simulink model "hw7_system"  (R2015a)
settings: Solver=ode3  StartTime=0.0  StopTime=20  FixedStep=.01  MaxStep=.01  MinStep=.01  RelTol=1e-3
settings Model: Creator=lbremer  LastModifiedBy=lbremer

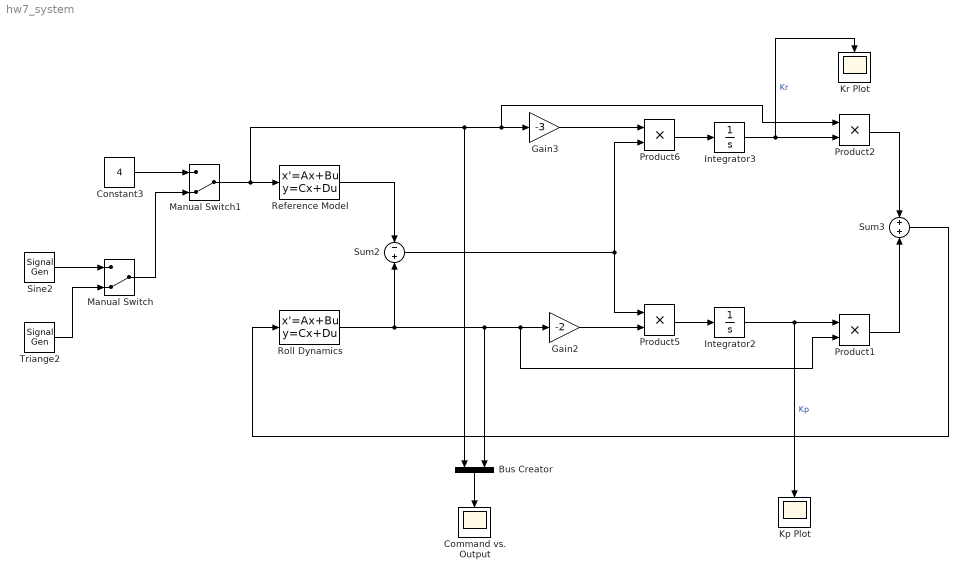
== system hw7_system ==
  Bus Creator : BusCreator  Inputs=2
  Command vs. Output : Scope
      settings: YMin=-1  YMax=1  SaveName=ScopeData4
  Constant3 : Constant  Value=4
  Gain2 : Gain  Gain=-2
  Gain3 : Gain  Gain=-3
  Integrator2 : Integrator
  Integrator3 : Integrator
  Kp Plot : Scope
      settings: YMin=-1  YMax=1
  "Kr Plot " : Scope
      settings: YMin=-1  YMax=1
  Manual Switch : ManualSwitch  CurrentSetting=0
  Manual Switch1 : ManualSwitch  CurrentSetting=0
  Product{1..2,5..6} (4 alike) : Product
  "Reference Model " : StateSpace  A=-6  B=6  D=0  X0=0
  "Roll Dynamics " : StateSpace  A=.7  B=3  D=0  X0=0
  Sine2 : SignalGenerator  Frequency=.5
  Sum2 : Sum  Inputs=-|+
  Sum3 : Sum  Inputs=+|+
  Triange2 : SignalGenerator  WaveForm=sawtooth  Frequency=2  Units=rad/sec
  wires:
  "Reference Model "/1 -> Sum2/1
  Sum2/1 -> Product5/1, Product6/2
  Gain2/1 -> Product5/2
  Product5/1 -> Integrator2/1
  Gain3/1 -> Product6/1
  Product6/1 -> Integrator3/1
  Sum3/1 -> "Roll Dynamics "/1
  Bus Creator/1 -> Command vs. Output/1
  Integrator2/1 -> Product1/1, Kp Plot/1  "Kp"
  "Roll Dynamics "/1 -> Product1/2, Gain2/1, Bus Creator/2, Sum2/2
  Product1/1 -> Sum3/2
  Integrator3/1 -> Product2/2, "Kr Plot "/1  "Kr"
  Manual Switch1/1 -> Bus Creator/1, Product2/1, Gain3/1, "Reference Model "/1
  Product2/1 -> Sum3/1
  Constant3/1 -> Manual Switch1/1
  Manual Switch/1 -> Manual Switch1/2
  Sine2/1 -> Manual Switch/1
  Triange2/1 -> Manual Switch/2
